simulink model "Aufgabenliste_digital_3_simulink"  (R2015a)
settings: Solver=ode4  StartTime=0.0  StopTime=10.0  FixedStep=0.001  RelTol=1e-3
libraries: cstblocks x2
settings Model: Creator=daniel  LastModifiedBy=daniel

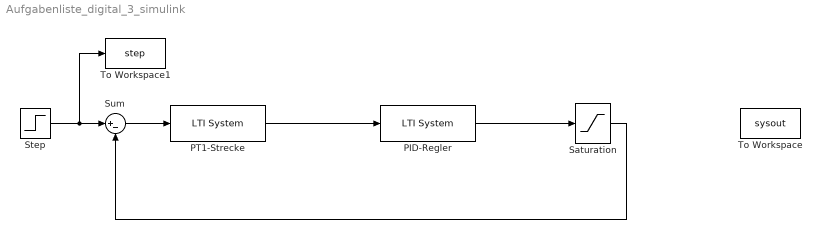
== system Aufgabenliste_digital_3_simulink ==
  PID-Regler : cstblocks/LTI System  sys=Regler  IC=[]
  PT1-Strecke : cstblocks/LTI System  sys=G  IC=[]
  Saturation : Saturate  UpperLimit=5  LowerLimit=-5
  Step : Step  After=5  SampleTime=0
  Sum : Sum  Inputs=|+-
  To Workspace : ToWorkspace  VariableName=sysout  SaveFormat=Structure With Time  SampleTime=-1
  To Workspace1 : ToWorkspace  VariableName=step  SaveFormat=Structure With Time  SampleTime=-1
  wires:
  PT1-Strecke/1 -> PID-Regler/1
  PID-Regler/1 -> Saturation/1
  Step/1 -> To Workspace1/1, Sum/1
  Sum/1 -> PT1-Strecke/1
  Saturation/1 -> Sum/2
